simulink model "QuadSim"  (R2023b)
settings: Solver=VariableStepAuto  StartTime=0.0  StopTime=4  RelTol=1e-4
libraries: robotcorelib x1
settings Model: Creator=baoth  LastModifiedBy=baoth
settings SolverCC: MaxConsecutiveMinStep=2
settings DebuggingCC: ModelReferenceExtraNoncontSigs=none

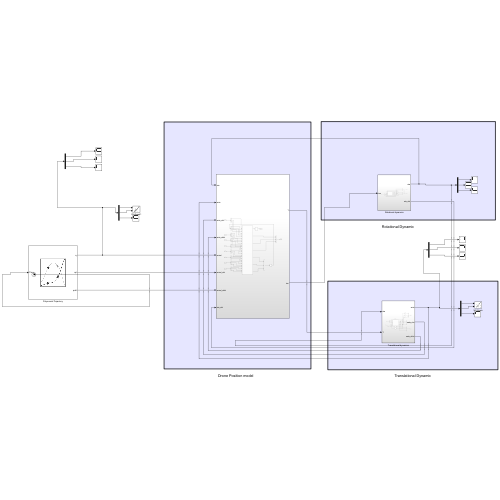
[thumbnail: Simulink's stored preview of the top-level diagram]
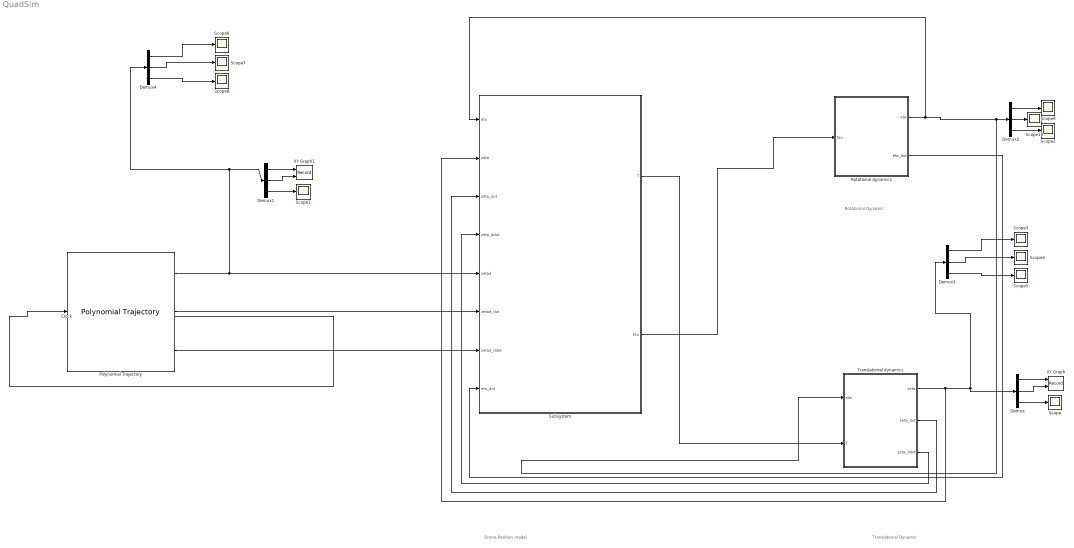
== system QuadSim ==
  note: Translational Dynamic
  note: Rotational Dynamic
  note: Drone Position model
  Clock : Clock
  Demux{,1..4} (5 alike) : Demux  Outputs=3
  Polynomial Trajectory : robotcorelib/Polynomial Trajectory  WaypointSource=Internal  Waypoints=[ 0 10 10 0 0; 0 0 10 10 0; 0 10 10 10 0 ]  TimePoints=[ 0, 1, 2, 3, 4 ]  TimeInterval=[ 1, 4 ]  Method=Quintic Polynomial  ParameterSource=Internal  VelocityBoundaryCondition=zeros( 3, 5 )  AccelerationBoundaryCondition=zeros( 3, 5 )  SimulateUsing=Interpreted execution
  Rotational dynamics : Subsystem
  Scope{,1..10} (11 alike) : Scope
  Subsystem : Subsystem
  Translational dynamics : Subsystem
  XY Graph : Record  FileSettingsInternal="{\"entries\":[{\"content\":{\"excelSettings\":{\"content\":{},\"type\":\"Streamout.ExcelSettings\"}},\"type\":\"Streamout.FileSettingStorage\",\"uuid\":\"\"}],\"packageUris\":[\"http:\\/\\/schema.mathworks.com\\/mf0\\/streamout_blocks\\/R2020a\"],\"version\":\"1.0\"}"  Layout=[1 1]  SignalsInternal="{\"entries\":[{\"content\":{\"signals\":[{\"content\":{\"blockPath\":[],\"dimensions\":[1],\"domain\":\"\",\"lineColor\":\"#a2142f\",\"plots\":[1],\"port\":1,\"signalID\":8,\"signalName\":\"Demux:1\"},\"type\":\"RecordBlkView.Signal\",\"uuid\":\"\"},{\"content\":{\"blockPath\":[],\"dimensions\":[1],\"domain\":\"\",\"lineColor\":\"#139fff\",\"plots\":[1],\"port\":2,\"signalID\":11,\"signalName\":\"Demux:2\"},\"type\":\"RecordBlkView.Signal\",\"uuid\":\"\"}]},\"type\":\"RecordBlkView.InputSignals\",\"uuid\":\"\"}],\"packageUris\":[\"http:\\/\\/schema.mathworks.com\\/mf0\\/streamout_blocks\\/R2020a\"],\"version\":\"1.0\"}"  VisualizationBindings="{\"xyplotplugin\":{\"info\":[{\"series\":[{\"bindingParametersList\":[{\"parameter\":\"X-Axis\",\"signalID\":8,\"signalName\":\"Demux:1\"},{\"parameter\":\"Y-Axis\",\"signalID\":11,\"signalName\":\"Demux:2\"}],\"seriesID\":37732}],\"subplotID\":1}]}}"  CompatibilityTag=XY
  XY Graph1 : Record  FileSettingsInternal="{\"entries\":[{\"content\":{\"excelSettings\":{\"content\":{},\"type\":\"Streamout.ExcelSettings\"}},\"type\":\"Streamout.FileSettingStorage\",\"uuid\":\"\"}],\"packageUris\":[\"http:\\/\\/schema.mathworks.com\\/mf0\\/streamout_blocks\\/R2020a\"],\"version\":\"1.0\"}"  Layout=[1 1]  SignalsInternal="{\"entries\":[{\"content\":{\"signals\":[{\"content\":{\"blockPath\":[],\"dimensions\":[1,1],\"domain\":\"\",\"lineColor\":\"#a2142f\",\"plots\":[1],\"port\":1,\"signalID\":16,\"signalName\":\"Demux1:1\"},\"type\":\"RecordBlkView.Signal\",\"uuid\":\"\"},{\"content\":{\"blockPath\":[],\"dimensions\":[1,1],\"domain\":\"\",\"lineColor\":\"#139fff\",\"plots\":[1],\"port\":2,\"signalID\":19,\"signalName\":\"Demux1:2\"},\"type\":\"RecordBlkView.Signal\",\"uuid\":\"\"}]},\"type\":\"RecordBlkView.InputSignals\",\"uuid\":\"\"}],\"packageUris\":[\"http:\\/\\/schema.mathworks.com\\/mf0\\/streamout_blocks\\/R2020a\"],\"version\":\"1.0\"}"  VisualizationBindings="{\"xyplotplugin\":{\"info\":[{\"series\":[{\"bindingParametersList\":[{\"parameter\":\"X-Axis\",\"signalID\":16,\"signalName\":\"Demux1:1\"},{\"parameter\":\"Y-Axis\",\"signalID\":19,\"signalName\":\"Demux1:2\"}],\"seriesID\":31099}],\"subplotID\":1}]}}"  CompatibilityTag=XY
  wires:
  Clock/1 -> Polynomial Trajectory/1
  Polynomial Trajectory/2 -> Subsystem/6(zetad_dot)
  Polynomial Trajectory/3 -> Subsystem/7(zetad_ddot)
  Translational dynamics/1(zeta) -> Subsystem/2(zeta), Demux3/1, Demux/1
  Translational dynamics/2(zeta_dot) -> Subsystem/3(zeta_dot)
  Translational dynamics/3(zeta_ddot) -> Subsystem/4(zeta_ddot)
  Subsystem/2(tau) -> Rotational dynamics/1(tau)
  Subsystem/1(T) -> Translational dynamics/2(T)
  Rotational dynamics/2(eta_dot) -> Subsystem/8(eta_dot)
  Demux/1 -> XY Graph/1
  Demux/2 -> XY Graph/2
  Demux/3 -> Scope/1
  Demux1/3 -> Scope1/1
  Demux1/2 -> XY Graph1/2
  Demux1/1 -> XY Graph1/1
  Demux2/3 -> Scope2/1
  Demux2/2 -> Scope10/1
  Demux2/1 -> Scope9/1
  Rotational dynamics/1(eta) -> Subsystem/1(eta), Demux2/1, Translational dynamics/1(eta)
  Demux3/1 -> Scope3/1
  Demux3/2 -> Scope4/1
  Demux3/3 -> Scope5/1
  Demux4/3 -> Scope8/1
  Demux4/2 -> Scope7/1
  Demux4/1 -> Scope6/1
  Polynomial Trajectory/1 -> Demux4/1, Demux1/1, Subsystem/5(zetad)

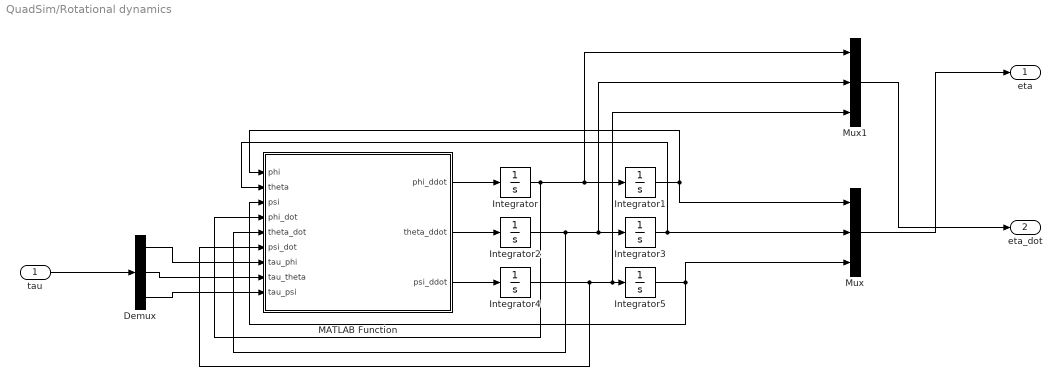
== system QuadSim/Rotational dynamics ==
  tau : Inport
  Demux : Demux  Outputs=3
  Integrator{,1..5} (6 alike) : Integrator
  MATLAB Function : MATLAB Function  TreatAsAtomicUnit=on
  Mux : Mux  Inputs=3
  Mux1 : Mux  Inputs=3
  eta : Outport
  eta_dot : Outport  Port=2
  wires:
  Integrator3/1 -> MATLAB Function/2(theta), Mux/2
  Integrator4/1 -> MATLAB Function/6(psi_dot), Mux1/3, Integrator5/1
  Integrator1/1 -> Mux/1, MATLAB Function/1(phi)
  Integrator/1 -> MATLAB Function/4(phi_dot), Mux1/1, Integrator1/1
  Integrator2/1 -> MATLAB Function/5(theta_dot), Integrator3/1, Mux1/2
  MATLAB Function/3(psi_ddot) -> Integrator4/1
  MATLAB Function/1(phi_ddot) -> Integrator/1
  Integrator5/1 -> Mux/3, MATLAB Function/3(psi)
  MATLAB Function/2(theta_ddot) -> Integrator2/1
  Mux/1 -> eta/1
  Mux1/1 -> eta_dot/1
  Demux/1 -> MATLAB Function/7(tau_phi)
  Demux/2 -> MATLAB Function/8(tau_theta)
  Demux/3 -> MATLAB Function/9(tau_psi)
  tau/1 -> Demux/1

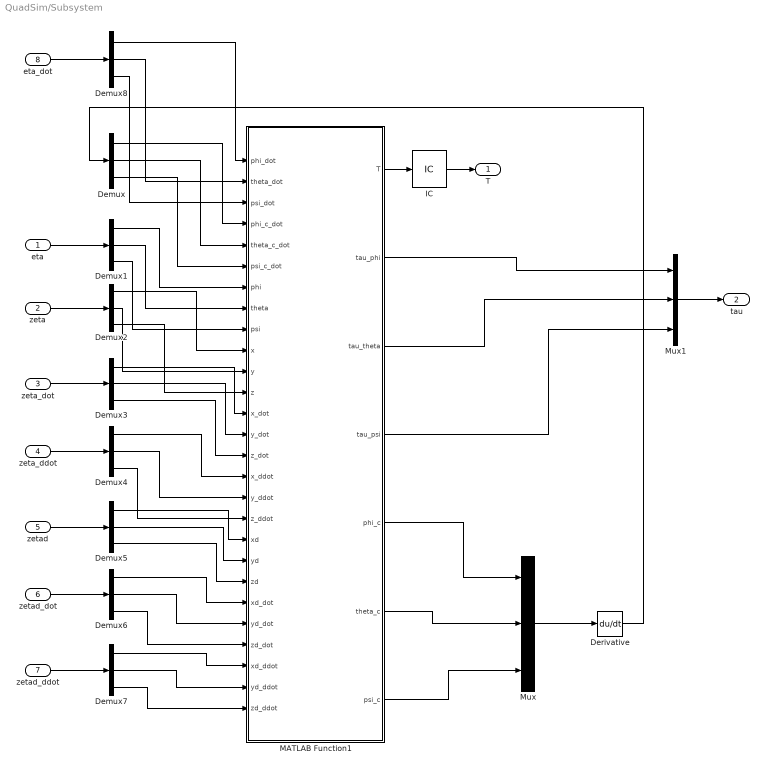
== system QuadSim/Subsystem ==
  eta : Inport
  zeta : Inport  Port=2
  zeta_dot : Inport  Port=3
  zeta_ddot : Inport  Port=4
  zetad : Inport  Port=5
  zetad_dot : Inport  Port=6
  zetad_ddot : Inport  Port=7
  eta_dot : Inport  Port=8
  Demux{,1..8} (9 alike) : Demux  Outputs=3
  Derivative : Derivative
  IC : InitialCondition  Value=0
  MATLAB Function1 : MATLAB Function  TreatAsAtomicUnit=on
  Mux : Mux  Inputs=3
  Mux1 : Mux  Inputs=3
  T : Outport
  tau : Outport  Port=2
  wires:
  zetad_ddot/1 -> Demux7/1
  Demux2/2 -> MATLAB Function1/11(y)
  Mux/1 -> Derivative/1
  Demux1/2 -> MATLAB Function1/8(theta)
  Mux1/1 -> tau/1
  MATLAB Function1/5(phi_c) -> Mux/1
  Derivative/1 -> Demux/1
  Demux1/1 -> MATLAB Function1/7(phi)
  Demux6/3 -> MATLAB Function1/24(zd_dot)
  zeta_dot/1 -> Demux3/1
  Demux3/3 -> MATLAB Function1/15(z_dot)
  zeta_ddot/1 -> Demux4/1
  Demux/2 -> MATLAB Function1/5(theta_c_dot)
  MATLAB Function1/2(tau_phi) -> Mux1/1
  Demux2/3 -> MATLAB Function1/12(z)
  Demux1/3 -> MATLAB Function1/9(psi)
  Demux4/3 -> MATLAB Function1/18(z_ddot)
  MATLAB Function1/3(tau_theta) -> Mux1/2
  Demux3/1 -> MATLAB Function1/13(x_dot)
  Demux5/3 -> MATLAB Function1/21(zd)
  Demux4/1 -> MATLAB Function1/16(x_ddot)
  eta/1 -> Demux1/1
  MATLAB Function1/1(T) -> IC/1
  Demux5/2 -> MATLAB Function1/20(yd)
  Demux2/1 -> MATLAB Function1/10(x)
  Demux6/2 -> MATLAB Function1/23(yd_dot)
  MATLAB Function1/6(theta_c) -> Mux/2
  Demux/3 -> MATLAB Function1/6(psi_c_dot)
  Demux7/2 -> MATLAB Function1/26(yd_ddot)
  Demux/1 -> MATLAB Function1/4(phi_c_dot)
  Demux5/1 -> MATLAB Function1/19(xd)
  MATLAB Function1/4(tau_psi) -> Mux1/3
  zetad_dot/1 -> Demux6/1
  Demux6/1 -> MATLAB Function1/22(xd_dot)
  Demux7/1 -> MATLAB Function1/25(xd_ddot)
  Demux4/2 -> MATLAB Function1/17(y_ddot)
  zetad/1 -> Demux5/1
  Demux3/2 -> MATLAB Function1/14(y_dot)
  zeta/1 -> Demux2/1
  Demux7/3 -> MATLAB Function1/27(zd_ddot)
  MATLAB Function1/7(psi_c) -> Mux/3
  Demux8/1 -> MATLAB Function1/1(phi_dot)
  Demux8/2 -> MATLAB Function1/2(theta_dot)
  Demux8/3 -> MATLAB Function1/3(psi_dot)
  eta_dot/1 -> Demux8/1
  IC/1 -> T/1

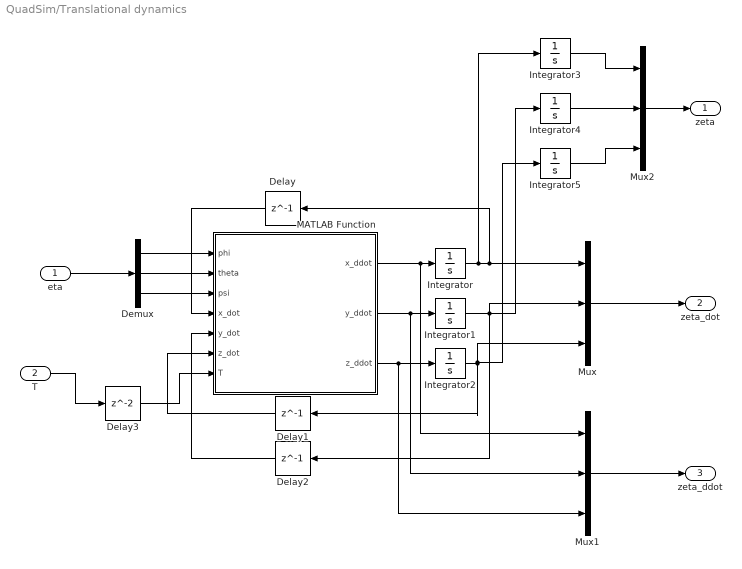
== system QuadSim/Translational dynamics ==
  eta : Inport
  T : Inport  Port=2
  Delay : Delay  DelayLength=1
  Delay1 : Delay  DelayLength=1
  Delay2 : Delay  DelayLength=1
  Delay3 : Delay
  Demux : Demux  Outputs=3
  Integrator{,1..5} (6 alike) : Integrator
  MATLAB Function : MATLAB Function  TreatAsAtomicUnit=on
  Mux : Mux  Inputs=3
  Mux1 : Mux  Inputs=3
  Mux2 : Mux  Inputs=3
  zeta : Outport
  zeta_dot : Outport  Port=2
  zeta_ddot : Outport  Port=3
  wires:
  Demux/1 -> MATLAB Function/1(phi)
  MATLAB Function/2(y_ddot) -> Integrator1/1, Mux1/2
  Integrator1/1 -> Integrator4/1, Mux/2, Delay2/1
  Integrator/1 -> Integrator3/1, Mux/1, Delay/1
  MATLAB Function/3(z_ddot) -> Integrator2/1, Mux1/3
  eta/1 -> Demux/1
  Demux/2 -> MATLAB Function/2(theta)
  Integrator2/1 -> Integrator5/1, Mux/3, Delay1/1
  MATLAB Function/1(x_ddot) -> Mux1/1, Integrator/1
  Demux/3 -> MATLAB Function/3(psi)
  Mux/1 -> zeta_dot/1
  Mux1/1 -> zeta_ddot/1
  Integrator3/1 -> Mux2/1
  Integrator4/1 -> Mux2/2
  Integrator5/1 -> Mux2/3
  Mux2/1 -> zeta/1
  Delay/1 -> MATLAB Function/4(x_dot)
  Delay1/1 -> MATLAB Function/6(z_dot)
  Delay2/1 -> MATLAB Function/5(y_dot)
  T/1 -> Delay3/1
  Delay3/1 -> MATLAB Function/7(T)

== matlab function QuadSim/Translational dynamics/MATLAB Function ==
  data: phi input; x_ddot output; theta input; psi input; x_dot input; y_dot input; z_dot input; T input; y_ddot output; z_ddot output
function [x_ddot, y_ddot, z_ddot] = fcn(phi, theta, psi, x_dot, y_dot, z_dot, T)

g = 9.81;
m = 0.468;
l = 0.225;
k = 2.980*10^-6;
b = 1.140*10^-7;
IM = 3.357*10^-5;

Ixx = 4.856*10^-3;
Iyy = 4.865*10^-3;
Izz = 8.801*10^-3;
Ax = 0.25;
Ay = 0.25;
Az = 0.25;

output = -g*[0;0;1] +...
    T/m*[cos(psi)*sin(theta)*cos(phi)+sin(psi)*sin(phi);...
            sin(psi)*sin(theta)*cos(phi) - cos(psi)*sin(phi);...
            cos(theta)*cos(phi)]+...
            -1/m*[Ax 0 0; 0 Ay 0; 0 0 Az]*[x_dot;y_dot;z_dot];
x_ddot = output(1);
y_ddot = output(2);
z_ddot = output(3);

== matlab function QuadSim/Rotational dynamics/MATLAB Function ==
  data: phi input; phi_ddot output; theta input; psi input; phi_dot input; theta_dot input; psi_dot input; tau_phi input; tau_theta input; tau_psi input; theta_ddot output; psi_ddot output
function [phi_ddot, theta_ddot, psi_ddot]  = fcn(phi, theta, psi, phi_dot, theta_dot, psi_dot, tau_phi, tau_theta, tau_psi)

g = 9.81;
m = 0.468;
l = 0.225;
k = 2.980*10^-6;
b = 1.140*10^-7;
IM = 3.357*10^-5;

Ixx = 4.856*10^-3;
Iyy = 4.865*10^-3;
Izz = 8.801*10^-3;
Ax = 0.25;
Ay = 0.25;
Az = 0.25;

J = [Ixx                0                                           -Ixx * sin(theta);
    0                   Iyy*cos(phi)^2 + Izz*sin(phi)^2             (Iyy - Izz)*cos(phi)*sin(phi)*cos(theta);
    -Ixx*sin(theta)     (Iyy - Izz)*cos(phi)*sin(phi)*cos(theta)    Ixx*sin(theta)^2+Iyy*sin(phi)^2*cos(theta)^2+Izz*cos(phi)^2*cos(theta)^2];


C = zeros(3,3);

C(1,1) = 0;
C(1,2) = (Iyy-Izz)*(theta_dot*cos(phi)*sin(phi)+psi_dot*sin(phi)^2*cos(theta)+...
    (Izz - Iyy)*psi_dot*cos(phi)^2*cos(theta)- Ixx*psi_dot*cos(theta));
C(1,3) = (Izz - Iyy)*psi_dot*cos(phi)*sin(phi)*cos(theta)^2;
C(2,1) = (Izz - Iyy)*(theta_dot*cos(phi)*sin(phi)+psi_dot*sin(phi)*cos(theta))+...
    (Iyy - Izz)*psi_dot*cos(phi)^2*cos(theta)+ Ixx*psi_dot*cos(theta);
C(2,2) = (Izz - Iyy)*phi_dot*cos(phi)*sin(phi);
C(2,3) = -Ixx*psi_dot*sin(theta)*cos(theta) + Iyy*psi_dot*sin(phi)^2*sin(theta)*cos(theta)+...
    Izz*psi_dot*cos(phi)^2*sin(theta)*cos(theta);
C(3,1) = (Iyy - Izz)*psi_dot*cos(theta)^2*sin(phi)*cos(phi) - Ixx*theta_dot*cos(theta);
C(3,2) = (Izz - Iyy)*(theta_dot*cos(phi)*sin(phi)*sin(theta)+phi_dot*sin(phi)^2*cos(theta))+...
    (Iyy - Izz)*phi_dot*cos(phi)^2*cos(theta) + Ixx*psi_dot*sin(theta)*cos(theta)-...
    Iyy*psi_dot*sin(phi)^2*sin(theta)*cos(theta) - Izz*psi_dot*cos(phi)^2*sin(theta)*cos(theta);
C(3,3) = (Iyy-Izz)*phi_dot*cos(phi)*sin(phi)*cos(theta)^2 - Iyy*theta_dot*sin(phi)^2*cos(theta)*sin(theta)-...
    Izz*theta_dot*cos(phi)^2*cos(theta)*sin(theta)*Ixx*theta_dot*cos(theta)*sin(theta);


eta_dot = [phi_dot; theta_dot; psi_dot];
tau = [tau_phi; tau_theta; tau_psi];

eta_ddot = inv(J)*(tau - C*eta_dot);

phi_ddot = eta_ddot(1);
theta_ddot = eta_ddot(2);
psi_ddot = eta_ddot(3);

== matlab function QuadSim/Subsystem/MATLAB Function1 ==
  data: phi_dot input; theta_dot input; psi_dot input; phi_c_dot input; T output; theta_c_dot input; psi_c_dot input; phi input; theta input; psi input; x input; y input; z input; x_dot input; y_dot input; z_dot input; x_ddot input; y_ddot input; z_ddot input; tau_phi output; tau_theta output; xd input; yd input; zd input; xd_dot input; yd_dot input; zd_dot input; xd_ddot input; yd_ddot input; zd_ddot input; tau_psi output; phi_c output; theta_c output; psi_c output
function [T, tau_phi, tau_theta, tau_psi, phi_c, theta_c, psi_c] = fcn(phi_dot, theta_dot, psi_dot, phi_c_dot, theta_c_dot, psi_c_dot, phi, theta, psi, x, y, z, x_dot, y_dot, z_dot, x_ddot, y_ddot, z_ddot, xd, yd, zd, xd_dot, yd_dot, zd_dot, xd_ddot, yd_ddot, zd_ddot)
g = 9.81;
m = 0.468;
l = 0.225;
k = 2.980*10^-6;
b = 1.140*10^-7;
IM = 3.357*10^-5;

Ixx = 4.856*10^-3;
Iyy = 4.865*10^-3;
Izz = 8.801*10^-3;
kxp = 4; kxd = 2; kxdd = 1;
kyp = 4; kyd = 2; kydd = 1;
kzp = 4; kzd = 2; kzdd = 1;
kphip = 8;  kphid = 2;
kthetap = 8; kthetad = 2;
kpsip = 10;  kpsid = 1;

dx = kxp * (xd - x) + kxd * (xd_dot - x_dot) + kxdd * (xd_ddot - x_ddot);
dy = kyp * (yd - y) + kyd * (yd_dot - y_dot) + kydd * (yd_ddot - y_ddot);
dz = kzp * (zd - z) + kzd * (zd_dot - z_dot) + kzdd * (zd_ddot - z_ddot);

phi_c = asin((dx*sin(psi)-dy*cos(psi)) / sqrt(dx^2+dy^2+(dz+g)^2));
theta_c = atan((dx*cos(psi)+dy*sin(psi)) / (dz+g));
psi_c = 0;
T = m * (dx*(sin(theta)*cos(psi)*cos(phi)+sin(psi)*sin(phi))+...
    + dy*(sin(theta)*sin(psi)*cos(phi)-cos(psi)*sin(phi))+...
    + (dz + g)*cos(theta)*cos(phi));

tau_phi = (kphip*(phi_c - phi) + kphid*(phi_c_dot - phi_dot))*Ixx;
tau_theta = (kthetap*(theta_c - theta) + kthetad*(theta_c_dot - theta_dot))*Iyy;
tau_psi = (kpsip*(psi_c - psi) + kpsid*(psi_c_dot - psi_dot))*Izz;
